simulink model "SimpleEngine"  (R2021b)
settings: Solver=VariableStepAuto  StartTime=0.0  StopTime=inf  RelTol=1e-3  EnableMultiTasking=on
model workspace (MAT data in the model file):
  AccPwrbp = Simulink.Parameter
  AccPwrbp.Value = [0 0]
  AccPwrbp.DataType = 'double'
  AccPwrbp.Complexity = 'real'
  AccPwrbp.Dimensions = [1 2]
  AccSpdbp = Simulink.Parameter
  AccSpdbp.Value = [300 750]
  AccSpdbp.DataType = 'double'
  AccSpdbp.Complexity = 'real'
  AccSpdbp.Dimensions = [1 2]
  BsfcAvg = Simulink.Parameter
  BsfcAvg.Value = 350
  BsfcAvg.DataType = 'auto'
  BsfcAvg.Complexity = 'real'
  BsfcAvg.Dimensions = [1 1]
  Cps = Simulink.Parameter
  Cps.Value = 2
  Cps.DataType = 'double'
  Cps.Complexity = 'real'
  Cps.Dimensions = [1 1]
  Lhv = Simulink.Parameter
  Lhv.Value = 46000000
  Lhv.DataType = 'double'
  Lhv.Complexity = 'real'
  Lhv.Dimensions = [1 1]
  Sg = Simulink.Parameter
  Sg.Value = 0.754
  Sg.DataType = 'auto'
  Sg.Complexity = 'real'
  Sg.Dimensions = [1 1]
  TimeCnstECP = Simulink.Parameter
  TimeCnstECP.Value = 0.125
  TimeCnstECP.DataType = 'double'
  TimeCnstECP.Complexity = 'real'
  TimeCnstECP.Dimensions = [1 1]
  TimeCnstEGR = Simulink.Parameter
  TimeCnstEGR.Value = 0.125
  TimeCnstEGR.DataType = 'double'
  TimeCnstEGR.Complexity = 'real'
  TimeCnstEGR.Dimensions = [1 1]
  TimeCnstETC = Simulink.Parameter
  TimeCnstETC.Value = 0.085
  TimeCnstETC.DataType = 'double'
  TimeCnstETC.Complexity = 'real'
  TimeCnstETC.Dimensions = [1 1]
  TimeCnstICP = Simulink.Parameter
  TimeCnstICP.Value = 0.125
  TimeCnstICP.DataType = 'double'
  TimeCnstICP.Complexity = 'real'
  TimeCnstICP.Dimensions = [1 1]
  TimeCnstIVL = Simulink.Parameter
  TimeCnstIVL.Value = 0.125
  TimeCnstIVL.DataType = 'double'
  TimeCnstIVL.Complexity = 'real'
  TimeCnstIVL.Dimensions = [1 1]
  TimeCnstMFA = Simulink.Parameter
  TimeCnstMFA.Value = 0.125
  TimeCnstMFA.DataType = 'double'
  TimeCnstMFA.Complexity = 'real'
  TimeCnstMFA.Dimensions = [1 1]
  TimeCnstSWVA = Simulink.Parameter
  TimeCnstSWVA.Value = 0.125
  TimeCnstSWVA.DataType = 'double'
  TimeCnstSWVA.Complexity = 'real'
  TimeCnstSWVA.Dimensions = [1 1]
  TimeCnstVCR = Simulink.Parameter
  TimeCnstVCR.Value = 0.125
  TimeCnstVCR.DataType = 'double'
  TimeCnstVCR.Complexity = 'real'
  TimeCnstVCR.Dimensions = [1 1]
  TimeCnstVGT = Simulink.Parameter
  TimeCnstVGT.Value = 0.15
  TimeCnstVGT.DataType = 'double'
  TimeCnstVGT.Complexity = 'real'
  TimeCnstVGT.Dimensions = [1 1]
  TimeCnstVIRL = Simulink.Parameter
  TimeCnstVIRL.Value = 0.125
  TimeCnstVIRL.DataType = 'double'
  TimeCnstVIRL.Complexity = 'real'
  TimeCnstVIRL.Dimensions = [1 1]
  TimeCnstWGA = Simulink.Parameter
  TimeCnstWGA.Value = 0.15
  TimeCnstWGA.DataType = 'double'
  TimeCnstWGA.Complexity = 'real'
  TimeCnstWGA.Dimensions = [1 1]
  f_tqmax = Simulink.Parameter
  f_tqmax.Value = [75.6797764808 75.6797764808 97.1736585381 116.840425992 152.210298827 175 174.998895206 174.999965201 175 175 175 175 175 175 175 175]
  f_tqmax.DataType = 'double'
  f_tqmax.Complexity = 'real'
  f_tqmax.Dimensions = [1 16]
  f_tqmax_n_bpt = Simulink.Parameter
  f_tqmax_n_bpt.Value = [0 750 1053.57142857 1357.14285714 1660.71428571 1964.28571429 2267.85714286 2571.42857143 2875 3178.57142857 3482.14285714 3785.71428571 4089.28571429 4392.85714286 4696.42857143 5000]
  f_tqmax_n_bpt.DataType = 'double'
  f_tqmax_n_bpt.Complexity = 'real'
  f_tqmax_n_bpt.Dimensions = [1 16]
libraries: autolibhevctrlrcommon x1, autolibpowerinfoutils x1, autolibsharedmappedengines x1, autolibutils x1
settings Model: DataDictionary=SimpleEngine.sldd  ModifiedByFormat=The MathWorks, Inc.  Creator=The MathWorks, Inc.  LastModifiedBy=The MathWorks, Inc.
settings SolverCC: AlgebraicLoopSolver=TrustRegion  DecoupledContinuousIntegration=on
settings DataIOCC: DSMLogging=off  ReturnWorkspaceOutputs=off
settings DebuggingCC: SFMachineParentedDataDiag=warning  ArithmeticOperatorsInVariantConditions=warning
settings SFSimCC: SimUseLocalCustomCode=off  CustomCodeUndefinedFunction=UseInterfaceOnly
settings RTWCC: RTWUseLocalCustomCode=off
settings CodeAppCC: StateflowObjectComments=on
settings GRTTargetCC: TargetLangStandard=C89/C90 (ANSI)
settings ConfigComp: CovMetricSettings=dsw  CovSaveCumulativeToWorkspaceVar=on  CovSaveSingleToWorkspaceVar=on  CovExternalEMLEnable=off
settings SimscapeCC: SimscapeNormalizeSystem=off  SimscapeNominalValues={1, 'bar'; 1, 'cm^3/s'; 1, 'bar*kg/s'; 1, 'kJ/kg'; 1, 'kW'}

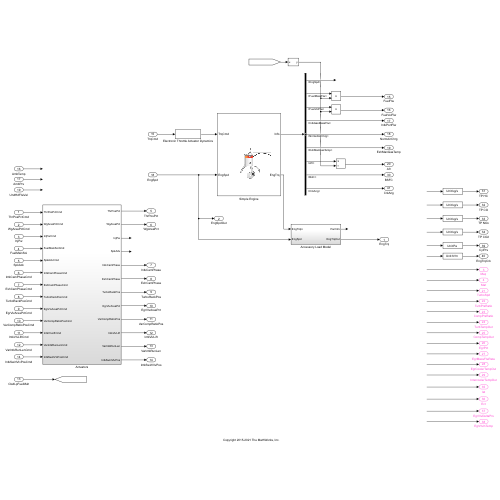
[thumbnail: Simulink's stored preview of the top-level diagram]
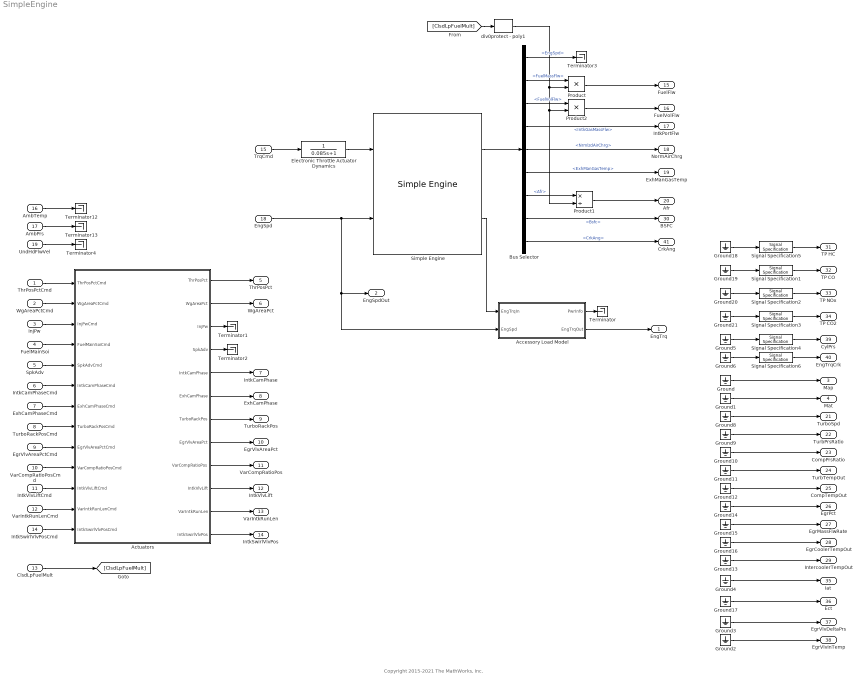
== system SimpleEngine ==
  note: Copyright 2015-2021 The MathWorks, Inc.
  ThrPosPctCmd : Inport
  WgAreaPctCmd : Inport  Port=2
  InjPw : Inport  Port=3
  FuelMainSoi : Inport  Port=4
  SpkAdv : Inport  Port=5
  IntkCamPhaseCmd : Inport  Port=6
  ExhCamPhaseCmd : Inport  Port=7
  TurboRackPosCmd : Inport  Port=8
  EgrVlvAreaPctCmd : Inport  Port=9
  VarCompRatioPosCmd : Inport  Port=10
  IntkVlvLiftCmd : Inport  Port=11
  VarIntkRunLenCmd : Inport  Port=12
  ClsdLpFuelMult : Inport  Port=13  Unit=1
  IntkSwirlVlvPosCmd : Inport  Port=14
  TrqCmd : Inport  Port=15  Unit=N*m
  AmbTemp : Inport  Port=16  Unit=K
  AmbPrs : Inport  Port=17  Unit=Pa
  EngSpd : Inport  Port=18  Interpolate=off
  UndHdFlwVel : Inport  Port=19  Unit=m/s
  Accessory Load Model : Subsystem
  Actuators : Subsystem
  Bus Selector : BusSelector  OutputSignals=EngSpd,FuelMassFlw,FuelVolFlw,IntkGasMassFlw,NrmlzdAirChrg,ExhManGasTemp,Afr,Bsfc,CrkAng
  Electronic Throttle Actuator Dynamics : TransferFcn  Denominator=[0.085 1]
  Ground{,1..6,8..21} (21 alike) : Ground
  Product : Product
  Product1 : Product  Inputs=*/
  Product2 : Product
  Signal Specification{1..3,5} (4 alike) : SignalSpecification  Unit=kg/s
  Signal Specification4 : SignalSpecification  Unit=Pa
  Signal Specification6 : SignalSpecification  Unit=N*m
  Simple Engine : autolibsharedmappedengines/Simple Engine  f_tqmax=f_tqmax  f_tqmax_n_bpt=f_tqmax_n_bpt  Lhv=Lhv  Sg=Sg  BsfcAvg=BsfcAvg  aMode=1
      settings: SourceProductBaseCode=PW,DR,MT,UV,VE
  Terminator{,1..4,12..13} (7 alike) : Terminator
  div0protect - poly1 : autolibutils/div0protect - poly  thresh=0.01  ZeroCross1=off  aMode=aMode
      settings: SourceProductBaseCode=PW,DR,MT,UV,VE
  EngTrq : Outport  Unit=N*m  VectorParamsAs1DForOutWhenUnconnected=off
  EngSpdOut : Outport  Port=2  VectorParamsAs1DForOutWhenUnconnected=off
  Map : Outport  Port=3  Unit=Pa  VectorParamsAs1DForOutWhenUnconnected=off
  Mat : Outport  Port=4  Unit=K  VectorParamsAs1DForOutWhenUnconnected=off
  ThrPosPct : Outport  Port=5  VectorParamsAs1DForOutWhenUnconnected=off
  WgAreaPct : Outport  Port=6  VectorParamsAs1DForOutWhenUnconnected=off
  IntkCamPhase : Outport  Port=7  VectorParamsAs1DForOutWhenUnconnected=off
  ExhCamPhase : Outport  Port=8  VectorParamsAs1DForOutWhenUnconnected=off
  TurboRackPos : Outport  Port=9  VectorParamsAs1DForOutWhenUnconnected=off
  EgrVlvAreaPct : Outport  Port=10  VectorParamsAs1DForOutWhenUnconnected=off
  VarCompRatioPos : Outport  Port=11  VectorParamsAs1DForOutWhenUnconnected=off
  IntkVlvLift : Outport  Port=12  VectorParamsAs1DForOutWhenUnconnected=off
  VarIntkRunLen : Outport  Port=13  VectorParamsAs1DForOutWhenUnconnected=off
  IntkSwirlVlvPos : Outport  Port=14  VectorParamsAs1DForOutWhenUnconnected=off
  FuelFlw : Outport  Port=15  Unit=kg/s  VectorParamsAs1DForOutWhenUnconnected=off
  FuelVolFlw : Outport  Port=16  Unit=m^3/s  VectorParamsAs1DForOutWhenUnconnected=off
  IntkPortFlw : Outport  Port=17  VectorParamsAs1DForOutWhenUnconnected=off
  NormAirChrg : Outport  Port=18  VectorParamsAs1DForOutWhenUnconnected=off
  ExhManGasTemp : Outport  Port=19  VectorParamsAs1DForOutWhenUnconnected=off
  Afr : Outport  Port=20  Unit=1  VectorParamsAs1DForOutWhenUnconnected=off
  TurboSpd : Outport  Port=21  Unit=rad/s  VectorParamsAs1DForOutWhenUnconnected=off
  TurbPrsRatio : Outport  Port=22  Unit=1  VectorParamsAs1DForOutWhenUnconnected=off
  CompPrsRatio : Outport  Port=23  Unit=1  VectorParamsAs1DForOutWhenUnconnected=off
  TurbTempOut : Outport  Port=24  Unit=K  VectorParamsAs1DForOutWhenUnconnected=off
  CompTempOut : Outport  Port=25  Unit=K  VectorParamsAs1DForOutWhenUnconnected=off
  EgrPct : Outport  Port=26  Unit=%  VectorParamsAs1DForOutWhenUnconnected=off
  EgrMassFlwRate : Outport  Port=27  Unit=kg/s  VectorParamsAs1DForOutWhenUnconnected=off
  EgrCoolerTempOut : Outport  Port=28  Unit=K  VectorParamsAs1DForOutWhenUnconnected=off
  IntercoolerTempOut : Outport  Port=29  Unit=K  VectorParamsAs1DForOutWhenUnconnected=off
  BSFC : Outport  Port=30  VectorParamsAs1DForOutWhenUnconnected=off
  TP HC : Outport  Port=31  VectorParamsAs1DForOutWhenUnconnected=off
  TP CO : Outport  Port=32  VectorParamsAs1DForOutWhenUnconnected=off
  TP NOx : Outport  Port=33  VectorParamsAs1DForOutWhenUnconnected=off
  TP CO2 : Outport  Port=34  VectorParamsAs1DForOutWhenUnconnected=off
  Iat : Outport  Port=35  Unit=K  VectorParamsAs1DForOutWhenUnconnected=off
  Ect : Outport  Port=36  Unit=K  VectorParamsAs1DForOutWhenUnconnected=off
  EgrVlvDeltaPrs : Outport  Port=37  Unit=Pa  VectorParamsAs1DForOutWhenUnconnected=off
  EgrVlvInTemp : Outport  Port=38  Unit=K  VectorParamsAs1DForOutWhenUnconnected=off
  CylPrs : Outport  Port=39  VectorParamsAs1DForOutWhenUnconnected=off
  EngTrqCrk : Outport  Port=40  VectorParamsAs1DForOutWhenUnconnected=off
  CrkAng : Outport  Port=41  VectorParamsAs1DForOutWhenUnconnected=off
  wires:
  ClsdLpFuelMult/1 -> [ClsdLpFuelMult]
  Bus Selector/9 -> CrkAng/1  "<CrkAng>"
  ThrPosPctCmd/1 -> Actuators/1(ThrPosPctCmd)
  Product/1 -> FuelFlw/1
  Ground21/1 -> Signal Specification3/1
  Bus Selector/6 -> ExhManGasTemp/1  "<ExhManGasTemp>"
  Ground20/1 -> Signal Specification2/1
  Accessory Load Model/2(EngTrqOut) -> EngTrq/1
  Ground19/1 -> Signal Specification1/1
  Ground12/1 -> CompTempOut/1
  Actuators/4(SpkAdv) -> Terminator2/1
  Bus Selector/1 -> Terminator3/1  "<EngSpd>"
  Ground18/1 -> Signal Specification5/1
  Actuators/1(ThrPosPct) -> ThrPosPct/1
  Ground9/1 -> TurbPrsRatio/1
  IntkCamPhaseCmd/1 -> Actuators/6(IntkCamPhaseCmd)
  Actuators/6(ExhCamPhase) -> ExhCamPhase/1
  Ground3/1 -> EgrVlvDeltaPrs/1
  [ClsdLpFuelMult] -> div0protect - poly1/1
  Bus Selector/5 -> NormAirChrg/1  "<NrmlzdAirChrg>"
  div0protect - poly1/1 -> Product2/2, Product1/2, Product/2
  Ground5/1 -> Signal Specification4/1
  Bus Selector/3 -> Product2/1  "<FuelVolFlw>"
  Actuators/5(IntkCamPhase) -> IntkCamPhase/1
  EngSpd/1 -> Simple Engine/2, Accessory Load Model/2(EngSpd), EngSpdOut/1
  SpkAdv/1 -> Actuators/5(SpkAdvCmd)
  Actuators/8(EgrVlvAreaPct) -> EgrVlvAreaPct/1
  Ground17/1 -> Ect/1
  Ground1/1 -> Mat/1
  Ground2/1 -> EgrVlvInTemp/1
  Ground6/1 -> Signal Specification6/1
  Actuators/9(VarCompRatioPos) -> VarCompRatioPos/1
  Ground10/1 -> CompPrsRatio/1
  Actuators/10(IntkVlvLift) -> IntkVlvLift/1
  ExhCamPhaseCmd/1 -> Actuators/7(ExhCamPhaseCmd)
  Accessory Load Model/1(PwrInfo) -> Terminator/1
  Ground/1 -> Map/1
  Actuators/3(InjPw) -> Terminator1/1
  Ground15/1 -> EgrMassFlwRate/1
  UndHdFlwVel/1 -> Terminator4/1
  IntkSwirlVlvPosCmd/1 -> Actuators/13(IntkSwirlVlvPosCmd)
  AmbPrs/1 -> Terminator13/1
  Actuators/11(VarIntkRunLen) -> VarIntkRunLen/1
  VarIntkRunLenCmd/1 -> Actuators/12(VarIntkRunLenCmd)
  Actuators/12(IntkSwirlVlvPos) -> IntkSwirlVlvPos/1
  Ground14/1 -> EgrPct/1
  IntkVlvLiftCmd/1 -> Actuators/11(IntkVlvLiftCmd)
  VarCompRatioPosCmd/1 -> Actuators/10(VarCompRatioPosCmd)
  Ground8/1 -> TurboSpd/1
  FuelMainSoi/1 -> Actuators/4(FuelMainSoiCmd)
  Ground4/1 -> Iat/1
  Bus Selector/8 -> BSFC/1  "<Bsfc>"
  Bus Selector/4 -> IntkPortFlw/1  "<IntkGasMassFlw>"
  Ground11/1 -> TurbTempOut/1
  Actuators/2(WgAreaPct) -> WgAreaPct/1
  TurboRackPosCmd/1 -> Actuators/8(TurboRackPosCmd)
  WgAreaPctCmd/1 -> Actuators/2(WgAreaPctCmd)
  Electronic Throttle Actuator Dynamics/1 -> Simple Engine/1
  Bus Selector/2 -> Product/1  "<FuelMassFlw>"
  Actuators/7(TurboRackPos) -> TurboRackPos/1
  TrqCmd/1 -> Electronic Throttle Actuator Dynamics/1
  Ground16/1 -> EgrCoolerTempOut/1
  AmbTemp/1 -> Terminator12/1
  Simple Engine/2 -> Accessory Load Model/1(EngTrqIn)
  Ground13/1 -> IntercoolerTempOut/1
  InjPw/1 -> Actuators/3(InjPwCmd)
  EgrVlvAreaPctCmd/1 -> Actuators/9(EgrVlvAreaPctCmd)
  Product1/1 -> Afr/1
  Product2/1 -> FuelVolFlw/1
  Simple Engine/1 -> Bus Selector/1
  Bus Selector/7 -> Product1/1  "<Afr>"
  Signal Specification5/1 -> TP HC/1
  Signal Specification1/1 -> TP CO/1
  Signal Specification2/1 -> TP NOx/1
  Signal Specification3/1 -> TP CO2/1
  Signal Specification4/1 -> CylPrs/1
  Signal Specification6/1 -> EngTrqCrk/1

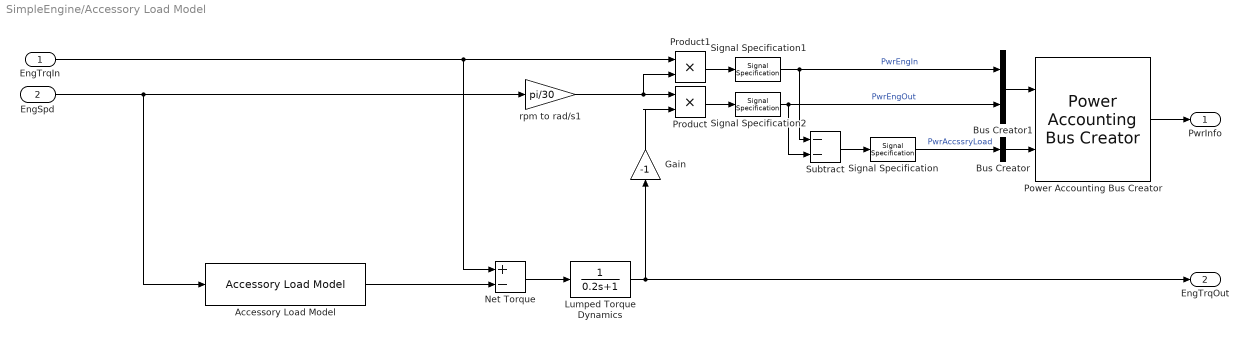
== system SimpleEngine/Accessory Load Model ==
  EngTrqIn : Inport
  EngSpd : Inport  Port=2
  Accessory Load Model : autolibhevctrlrcommon/Accessory Load Model  AccPwrTbl=[0 0]  AccSpdBpts=[300 750]
      settings: SourceProductBaseCode=PW
  Bus Creator : BusCreator  Inputs=1
  Bus Creator1 : BusCreator  Inputs=2
  Gain : Gain  Gain=-1
  Lumped Torque Dynamics : TransferFcn  Denominator=[0.2 1]
  Net Torque : Sum  Inputs=+-
  Power Accounting Bus Creator : autolibpowerinfoutils/Power Accounting Bus Creator  AssctBlkSelPopup=Parent  RefBlkName='libraryname/blkname'  PwrTrnsfrdCheckBox=on  PwrNotTrnsfrdCheckBox=on  PwrStoredCheckBox=off  aMode=aMode
      settings: SourceProductBaseCode=PW,DR,MT,UV,VE
  Product : Product
  Product1 : Product
  Signal Specification : SignalSpecification  Unit=W
  Signal Specification1 : SignalSpecification  Unit=W
  Signal Specification2 : SignalSpecification  Unit=W
  Subtract : Sum  Inputs=--
  rpm to rad/s1 : Gain  Gain=pi/30
  PwrInfo : Outport  VectorParamsAs1DForOutWhenUnconnected=off
  EngTrqOut : Outport  Port=2  Unit=N*m  VectorParamsAs1DForOutWhenUnconnected=off
  wires:
  Accessory Load Model/1 -> Net Torque/2
  EngSpd/1 -> Accessory Load Model/1, rpm to rad/s1/1
  Lumped Torque Dynamics/1 -> EngTrqOut/1, Gain/1
  Net Torque/1 -> Lumped Torque Dynamics/1
  Bus Creator/1 -> Power Accounting Bus Creator/2
  Bus Creator1/1 -> Power Accounting Bus Creator/1
  EngTrqIn/1 -> Product1/1, Net Torque/1
  Subtract/1 -> Signal Specification/1
  Signal Specification/1 -> Bus Creator/1  "PwrAccssryLoad"
  Power Accounting Bus Creator/1 -> PwrInfo/1
  Product/1 -> Signal Specification2/1
  Product1/1 -> Signal Specification1/1
  rpm to rad/s1/1 -> Product1/2, Product/1
  Signal Specification1/1 -> Subtract/1, Bus Creator1/1  "PwrEngIn"
  Signal Specification2/1 -> Subtract/2, Bus Creator1/2  "PwrEngOut"
  Gain/1 -> Product/2

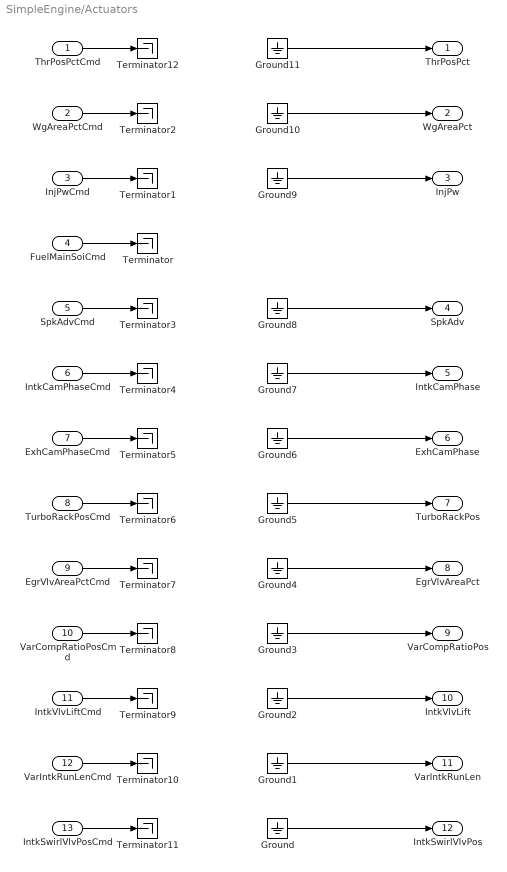
== system SimpleEngine/Actuators ==
  ThrPosPctCmd : Inport  Unit=%
  WgAreaPctCmd : Inport  Port=2  Unit=%
  InjPwCmd : Inport  Port=3  Unit=ms
  FuelMainSoiCmd : Inport  Port=4  Unit=deg
  SpkAdvCmd : Inport  Port=5  Unit=deg
  IntkCamPhaseCmd : Inport  Port=6  Unit=deg
  ExhCamPhaseCmd : Inport  Port=7  Unit=deg
  TurboRackPosCmd : Inport  Port=8  Unit=1
  EgrVlvAreaPctCmd : Inport  Port=9  Unit=%
  VarCompRatioPosCmd : Inport  Port=10
  IntkVlvLiftCmd : Inport  Port=11
  VarIntkRunLenCmd : Inport  Port=12
  IntkSwirlVlvPosCmd : Inport  Port=13
  Ground{,1..11} (12 alike) : Ground
  Terminator{,1..12} (13 alike) : Terminator
  ThrPosPct : Outport  Unit=%  VectorParamsAs1DForOutWhenUnconnected=off
  WgAreaPct : Outport  Port=2  Unit=%  VectorParamsAs1DForOutWhenUnconnected=off
  InjPw : Outport  Port=3  VectorParamsAs1DForOutWhenUnconnected=off
  SpkAdv : Outport  Port=4  VectorParamsAs1DForOutWhenUnconnected=off
  IntkCamPhase : Outport  Port=5  Unit=deg  VectorParamsAs1DForOutWhenUnconnected=off
  ExhCamPhase : Outport  Port=6  Unit=deg  VectorParamsAs1DForOutWhenUnconnected=off
  TurboRackPos : Outport  Port=7  Unit=1  VectorParamsAs1DForOutWhenUnconnected=off
  EgrVlvAreaPct : Outport  Port=8  Unit=%  VectorParamsAs1DForOutWhenUnconnected=off
  VarCompRatioPos : Outport  Port=9  VectorParamsAs1DForOutWhenUnconnected=off
  IntkVlvLift : Outport  Port=10  VectorParamsAs1DForOutWhenUnconnected=off
  VarIntkRunLen : Outport  Port=11  VectorParamsAs1DForOutWhenUnconnected=off
  IntkSwirlVlvPos : Outport  Port=12  VectorParamsAs1DForOutWhenUnconnected=off
  wires:
  Ground3/1 -> VarCompRatioPos/1
  Ground2/1 -> IntkVlvLift/1
  Ground1/1 -> VarIntkRunLen/1
  Ground/1 -> IntkSwirlVlvPos/1
  Ground7/1 -> IntkCamPhase/1
  Ground6/1 -> ExhCamPhase/1
  Ground10/1 -> WgAreaPct/1
  Ground11/1 -> ThrPosPct/1
  FuelMainSoiCmd/1 -> Terminator/1
  IntkVlvLiftCmd/1 -> Terminator9/1
  IntkSwirlVlvPosCmd/1 -> Terminator11/1
  WgAreaPctCmd/1 -> Terminator2/1
  ThrPosPctCmd/1 -> Terminator12/1
  ExhCamPhaseCmd/1 -> Terminator5/1
  IntkCamPhaseCmd/1 -> Terminator4/1
  VarCompRatioPosCmd/1 -> Terminator8/1
  VarIntkRunLenCmd/1 -> Terminator10/1
  InjPwCmd/1 -> Terminator1/1
  Ground5/1 -> TurboRackPos/1
  Ground4/1 -> EgrVlvAreaPct/1
  TurboRackPosCmd/1 -> Terminator6/1
  EgrVlvAreaPctCmd/1 -> Terminator7/1
  SpkAdvCmd/1 -> Terminator3/1
  Ground8/1 -> SpkAdv/1
  Ground9/1 -> InjPw/1
